simulink model "task3"  (R2021a)
settings: Solver=VariableStepAuto  StartTime=0.0  StopTime=10.0  RelTol=1e-3
undefined symbols (not defined in the file or in its folder): i
libraries: dspxfrm3 x3
settings Model: Creator=Nadir  LastModifiedBy=Nadir

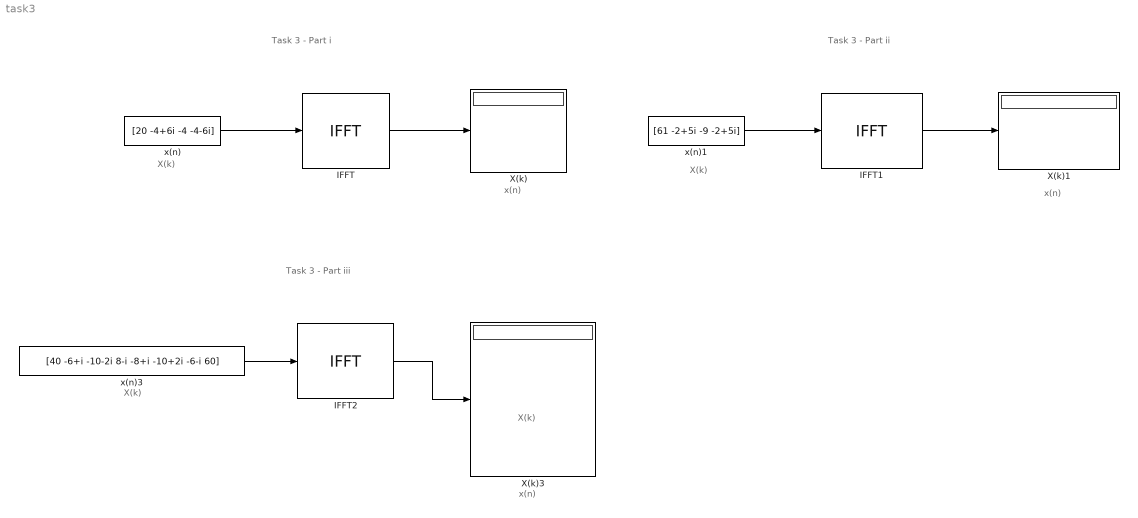
== system task3 ==
  note: x(n)
  note: x(n)
  note: Task 3 - Part i
  note: x(n)
  note: X(k)
  note: X(k)
  note: X(k)
  note: Task 3 - Part ii
  note: Task 3 - Part iii
  note: X(k)
  IFFT : dspxfrm3/IFFT  FFTImplementation=Auto  CompMethod=Table lookup  TableOpt=NEW  TableOptActive=Speed  BitRevOrder=off  cs_in=off  Normalize=on  InheritFFTLength=on  FFTLength=64  WrapInput=on  mode=Complex  outSamplingMode=Sample based  roundingMode=Floor  overflowMode=off  firstCoeffDataTypeStr=Inherit: Same word length as input  firstCoeffLastDataTypeStr=Inherit: Same word length as input  outputMin=[]  outputMax=[]
  IFFT1 : dspxfrm3/IFFT  FFTImplementation=Auto  CompMethod=Table lookup  TableOpt=NEW  TableOptActive=Speed  BitRevOrder=off  cs_in=off  Normalize=on  InheritFFTLength=on  FFTLength=64  WrapInput=on  mode=Complex  outSamplingMode=Sample based  roundingMode=Floor  overflowMode=off  firstCoeffDataTypeStr=Inherit: Same word length as input  firstCoeffLastDataTypeStr=Inherit: Same word length as input  outputMin=[]  outputMax=[]
  IFFT2 : dspxfrm3/IFFT  FFTImplementation=Auto  CompMethod=Table lookup  TableOpt=NEW  TableOptActive=Speed  BitRevOrder=off  cs_in=off  Normalize=on  InheritFFTLength=on  FFTLength=64  WrapInput=on  mode=Complex  outSamplingMode=Sample based  roundingMode=Floor  overflowMode=off  firstCoeffDataTypeStr=Inherit: Same word length as input  firstCoeffLastDataTypeStr=Inherit: Same word length as input  outputMin=[]  outputMax=[]
  X(k) : Display
  X(k)1 : Display
  X(k)3 : Display
  x(n) : Constant  Value=[20 -4+6i -4 -4-6i]
  x(n)1 : Constant  Value=[61 -2+5i -9 -2+5i]
  x(n)3 : Constant  Value=[40 -6+i -10-2i 8-i -8+i -10+2i -6-i 60]
  wires:
  IFFT/1 -> X(k)/1
  x(n)3/1 -> IFFT2/1
  x(n)1/1 -> IFFT1/1
  x(n)/1 -> IFFT/1
  IFFT1/1 -> X(k)1/1
  IFFT2/1 -> X(k)3/1
